simulink model "trackingControl"  (R2018a)
settings: Solver=VariableStepAuto  StartTime=0.0  StopTime=500  RelTol=1e-3
values from neighbouring files (symbols this model uses):
  K1 = [K(1,1) K(1,2);K(2,1) K(2,2)]    [trackingControlScript.m]
  K2 = [K(1,3) K(1,4);K(2,3) K(2,4)]    [trackingControlScript.m]
settings Model: Creator=Haydar  LastModifiedBy=Haydar

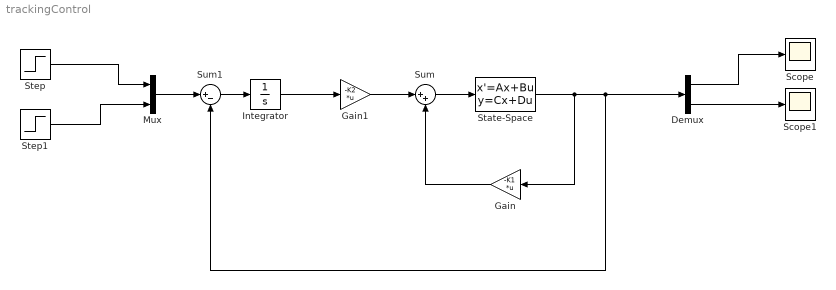
== system trackingControl ==
  Demux : Demux  Outputs=2
  Gain : Gain  Gain=-K1  Multiplication=Matrix(K*u)
  Gain1 : Gain  Gain=-K2  Multiplication=Matrix(K*u)
  Integrator : Integrator
  Mux : Mux  Inputs=2
  Scope : Scope
  Scope1 : Scope
  State-Space : StateSpace  A=[-0.01 0;0 -0.02]  B=[0.01 0;-0.03 0.04]  C=[1 0;0 1]  D=[0 0;0 0]  InitialCondition=0
  Step : Step  Time=0  After=10  SampleTime=0
  Step1 : Step  Time=0  After=2  SampleTime=0
  Sum : Sum  Inputs=|++
  Sum1 : Sum  Inputs=|+-
  wires:
  Sum/1 -> State-Space/1
  Step/1 -> Mux/1
  Step1/1 -> Mux/2
  Mux/1 -> Sum1/1
  Gain/1 -> Sum/2
  Sum1/1 -> Integrator/1
  Integrator/1 -> Gain1/1
  State-Space/1 -> Gain/1, Sum1/2, Demux/1
  Gain1/1 -> Sum/1
  Demux/1 -> Scope/1
  Demux/2 -> Scope1/1
